simulink model "FS_FD1"  (R2021a)
settings: Solver=FixedStepAuto  StartTime=0.0  StopTime=inf  RelTol=1e-3
values from neighbouring files (symbols this model uses):
  waypoints = [0 0 0.089 0.468 1.137 1.887 2.636 3.385 4.128 4.865 5.608 6.345 ... (52 elements, 26x2)]    [waypoints_straight_corridor.mat]
undefined symbols (not defined in the file or in its folder): Angular, Linear
libraries: robotlib x5, robotalgslib x1, robotcorelib x1
settings Model: Creator=ACER  LastModifiedBy=tarun
settings OptimizationCC: EnhancedBackFolding=on  PassReuseOutputArgsAs=Individual arguments  ZeroExternalMemoryAtStartup=off  ZeroInternalMemoryAtStartup=off  MaxStackSize=64  OptimizeBlockOrder=speed  DifferentSizesBufferReuse=on  OptimizationCustomize=off  EfficientTunableParamExpr=on
settings DebuggingCC: ParameterTunabilityLossMsg=error
settings HardwareCC: ProdBitPerPointer=32  ProdBitPerSizeT=32  ProdBitPerPtrDiffT=32  ProdLargestAtomicFloat=None  ProdIntDivRoundTo=Undefined  ProdEndianess=Unspecified  ProdWordSize=32  ProdHWDeviceType=Generic->Unspecified (assume 32-bit Generic)
settings SFSimCC: MATLABDynamicMemAlloc=off
settings RTWCC: SystemTargetFile=ert.tlc  HardwareBoard=Robot Operating System (ROS)  TLCOptions="-aInlineSetEventsForThisBaseRateFcn=TLC_FALSE -aSuppressMultiTaskScheduler=TLC_FALSE  -aRateBasedStepFcn=0"  TemplateMakefile=ert_default_tmf  Toolchain=Catkin  TargetLang=C++
settings CodeAppCC: ForceParamTrailComments=on  IgnoreCustomStorageClasses=off  OperatorAnnotations=on  SimulinkDataObjDesc=on  SFDataObjDesc=on  InsertBlockDesc=on

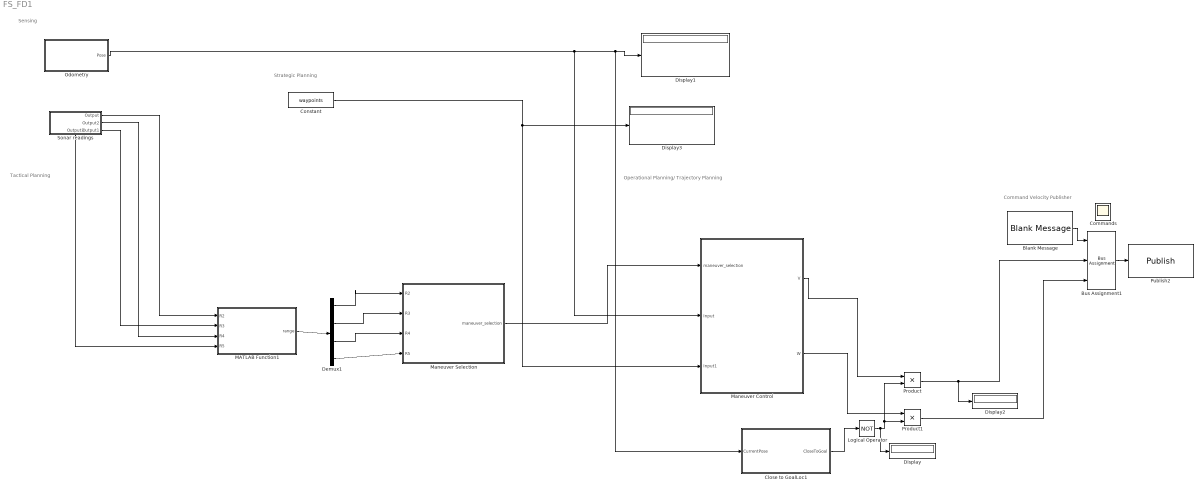
== system FS_FD1 ==
  note: Operational Planning/ Trajectory Planning
  note: Sensing
  note: Command Velocity Publisher
  note: Tactical Planning
  note: Strategic Planning
  Blank Message : robotlib/Blank Message  messageClass=Message  entityType=geometry_msgs/Twist  messageType=geometry_msgs/Twist  SampleTime=inf  legacyBusStruct=off
  Bus Assignment1 : BusAssignment  DialogController=Simulink.DDGSource_BusAssignment  AssignedSignals=Linear.X,Angular.Z
  Close to GoalLoc1 : Subsystem
  Commands : Scope  NumInputPorts=2
  Constant : Constant  Value=waypoints
  Demux1 : Demux
  Display{,1..3} (4 alike) : Display
  Logical Operator : Logic  Operator=NOT  AllPortsSameDT=off  OutDataTypeStr=boolean
  MATLAB Function1 : MATLAB Function  TreatAsAtomicUnit=on
  Maneuver Control : Subsystem
  Maneuver Selection : MATLAB Function  TreatAsAtomicUnit=on
  Odometry : Subsystem
  Product : Product
  Product1 : Product
  Publish2 : robotlib/Publish  topicSource=Select from ROS network  topic=/RosAria/cmd_vel  messageType=geometry_msgs/Twist  legacyBusStruct=off  messageQueueLength=105
  Sonar readings : Subsystem
      settings: PortSchema="{\"entries\":[{\"content\":{\"sides\":[{\"content\":{\"connectorIds\":[]},\"type\":\"ConnectorPlacement.EquallySpacedRectSide\",\"uuid\":\"cc9797a8-6551-4cc5-a464-2dfca9ae896a\"},{\"content\":{\"connectorIds\":[\"Out1\",\"Out2\",\"Out3\"],\"side\":\"RIGHT\"},\"type\":\"ConnectorPlacement.EquallySpacedRectSide\",\"uuid\":\"b2fd65e6-17ea-4988-b701-3713dcbefee6\"},{\"content\":{\"connectorIds\":[],\"side\":\"TOP\"},\"type\":\"ConnectorPlacement.EquallySpacedRectSide\",\"uuid\":\"23b966e9-18b1-4c56-9e9a-dc80dff313c9\"},{\"content\":{\"connectorIds\":[\"Out4\"],\"side\":\"BOTTOM\"},\"type\":\"ConnectorPlacement.EquallySpacedRectSide\",\"uuid\":\"b956123c-e71d-4c0e-8fc7-9c19c9412571\"}]},\"type\":\"ConnectorPlacement.EquallySpacedConnector\",\"uuid\":\"775a63bd-a867-418c-8661-cbcc6b0161f7\"}],\"packageUris\":[\"http://schema.mathworks.com/mf0/Connector/R2020b\"],\"version\":\"1.0\"}"
  wires:
  Constant/1 -> Maneuver Control/3(Input1), Display3/1
  Maneuver Control/1(V) -> Product/1
  Blank Message/1 -> Bus Assignment1/1
  Maneuver Selection/1(maneuver_selection) -> Maneuver Control/1(maneuver_selection)
  Bus Assignment1/1 -> Publish2/1
  Maneuver Control/2(W) -> Product1/1
  MATLAB Function1/1(range) -> Demux1/1
  Demux1/1 -> Maneuver Selection/1(R2)
  Demux1/2 -> Maneuver Selection/2(R3)
  Demux1/3 -> Maneuver Selection/3(R4)
  Demux1/4 -> Maneuver Selection/4(R5)
  Sonar readings/1(Output) -> MATLAB Function1/1(R2)
  Sonar readings/3(Output1) -> MATLAB Function1/2(R3)
  Sonar readings/2(Output2) -> MATLAB Function1/3(R4)
  Sonar readings/4(Output3) -> MATLAB Function1/4(R5)
  Odometry/1(Pose) -> Display1/1, Close to GoalLoc1/1(CurrentPose), Maneuver Control/2(Input)
  Close to GoalLoc1/1(CloseToGoal) -> Logical Operator/1
  Logical Operator/1 -> Display/1, Product1/2, Product/2
  Product/1 -> Display2/1, Bus Assignment1/2
  Product1/1 -> Bus Assignment1/3

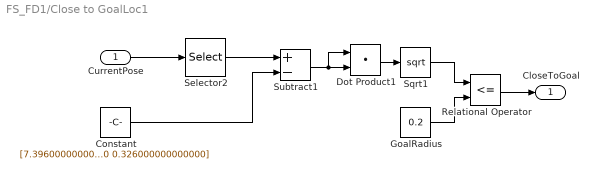
== system FS_FD1/Close to GoalLoc1 ==
  CurrentPose : Inport
  Constant : Constant  Value="[7.39600000000000\t0.326000000000000]"
  Dot Product1 : DotProduct  InputSameDT=on  OutDataTypeStr=Inherit: Inherit via internal rule
  GoalRadius : Constant  Value=0.2
  Relational Operator : RelationalOperator  Operator=<=  OutDataTypeStr=boolean  RndMeth=Simplest
  Selector2 : Selector  InputPortWidth=3  IndexOptions=Index vector (dialog)  Indices=[1 2]  OutputSizes=1
  Sqrt1 : Sqrt  SaturateOnIntegerOverflow=on
  Subtract1 : Sum  Inputs=+-
  CloseToGoal : Outport  VectorParamsAs1DForOutWhenUnconnected=off
  wires:
  Dot Product1/1 -> Sqrt1/1
  Subtract1/1 -> Dot Product1/1, Dot Product1/2
  Selector2/1 -> Subtract1/1
  Constant/1 -> Subtract1/2
  Sqrt1/1 -> Relational Operator/1
  GoalRadius/1 -> Relational Operator/2
  CurrentPose/1 -> Selector2/1
  Relational Operator/1 -> CloseToGoal/1

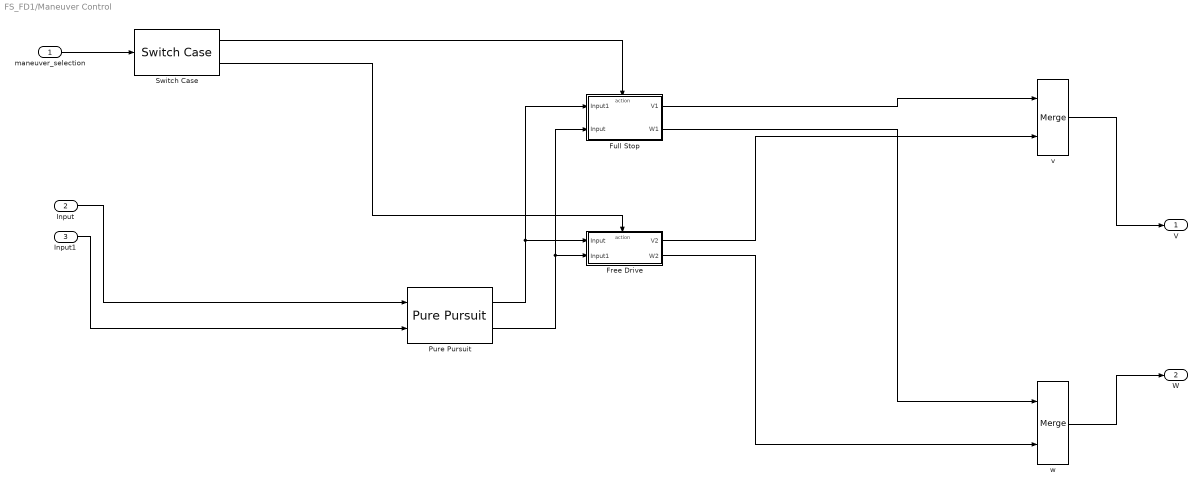
== system FS_FD1/Maneuver Control ==
  maneuver_selection : Inport
  Input : Inport  Port=2
  Input1 : Inport  Port=3
  Free Drive : Subsystem  TreatAsAtomicUnit=on
  Full Stop : Subsystem  TreatAsAtomicUnit=on
  Pure Pursuit : robotalgslib/Pure Pursuit  DesiredLinearVelocity=0.5  MaxAngularVelocity=0.8  LookaheadDistance=0.6  TargetDirPort=off  SimulateUsing=Code generation
  Switch Case : SwitchCase  CaseConditions={1,2}  ShowDefaultCase=off
  v : Merge
  w : Merge
  V : Outport
  W : Outport  Port=2
  wires:
  maneuver_selection/1 -> Switch Case/1
  Switch Case/1 -> Full Stop/Action
  Pure Pursuit/2 -> Full Stop/2(Input), Free Drive/2(Input1)
  Pure Pursuit/1 -> Full Stop/1(Input1), Free Drive/1(Input)
  Input1/1 -> Pure Pursuit/2
  Input/1 -> Pure Pursuit/1
  Free Drive/1(V2) -> v/2
  w/1 -> W/1
  v/1 -> V/1
  Switch Case/2 -> Free Drive/Action
  Full Stop/1(V1) -> v/1
  Full Stop/2(W1) -> w/1
  Free Drive/2(W2) -> w/2

== system FS_FD1/Odometry ==
  note: Generate a pose vector (x, y, theta) from X, Y, and quaternion data
  Bus Selector1 : BusSelector  OutputSignals=Pose.Pose.Position.X,Pose.Pose.Position.Y,Pose.Pose.Orientation.W,Pose.Pose.Orientation.X,Pose.Pose.Orientation.Y,Pose.Pose.Orientation.Z
  Coordinate Transformation Conversion : robotcorelib/Coordinate Transformation Conversion  InputRepresentation=Quaternion  InputEulerSequence=ZYX  ShowTrVecInputPort=on  OutputRepresentation=Euler Angles  OutputEulerSequence=ZYX  ShowTrVecOutputPort=on  SimulateUsing=Interpreted execution
      settings: SourceProductBaseCode=NV,RO,RR,UV
  Mux1 : Mux  Inputs=2
  Mux2 : Mux  Inputs=2
  Selector2 : Selector  InputPortWidth=3  IndexOptions=Index vector (dialog)  Indices=1  OutputSizes=1
  Subscribe1 : robotlib/Subscribe  topicSource=Select from ROS network  topic=/RosAria/pose  messageType=nav_msgs/Odometry  SampleTime=0.05  legacyBusStruct=off  messageQueueLength=51
  Terminator : Terminator
  Vector Concatenate : Concatenate  NumInputs=4
  Pose : Outport  VectorParamsAs1DForOutWhenUnconnected=off
  wires:
  Vector Concatenate/1 -> Coordinate Transformation Conversion/1
  Coordinate Transformation Conversion/1 -> Selector2/1
  Mux1/1 -> Mux2/1
  Selector2/1 -> Mux2/2
  Mux2/1 -> Pose/1
  Bus Selector1/6 -> Vector Concatenate/4  "<Z>"
  Bus Selector1/1 -> Mux1/1  "<X>"
  Bus Selector1/4 -> Vector Concatenate/2  "<X>"
  Bus Selector1/2 -> Mux1/2  "<Y>"
  Bus Selector1/5 -> Vector Concatenate/3  "<Y>"
  Subscribe1/2 -> Bus Selector1/1
  Bus Selector1/3 -> Vector Concatenate/1  "<W>"
  Subscribe1/1 -> Terminator/1

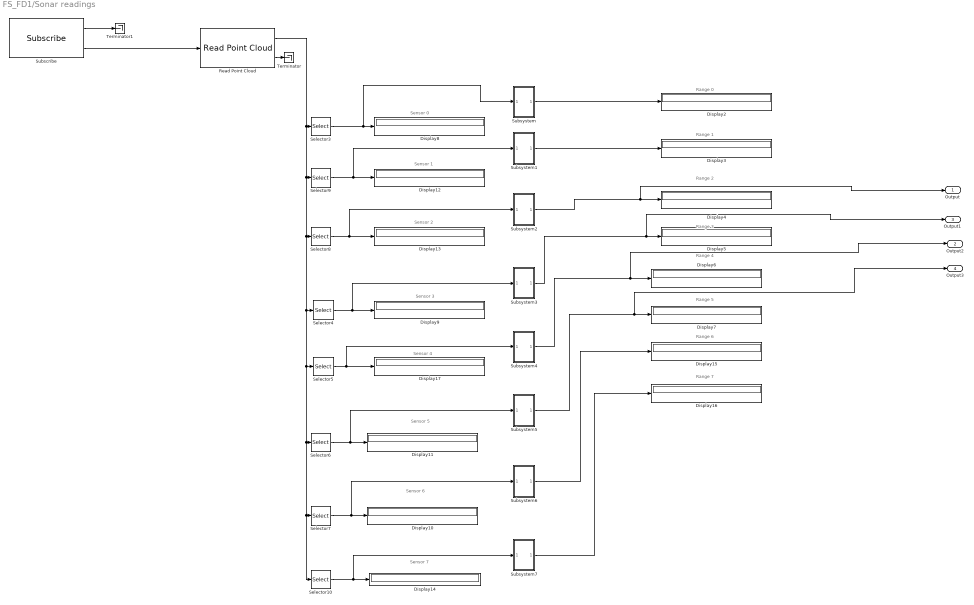
== system FS_FD1/Sonar readings ==
  note: Range 3
  note: Range 5
  note: Sensor 7
  note: Sensor 6
  note: Range 0
  note: Sensor 0
  note: Range 2
  note: Range 4
  note: Range 6
  note: Range 7
  note: Sensor 2
  note: Sensor 3
  note: Sensor 5
  note: Range 1
  note: Sensor 4
  note: Sensor 1
  Display{2..17} (16 alike) : Display
  Read Point Cloud : robotlib/Read Point Cloud  MaximumPointCloudSize=[8, 1]  PreserveStructure=off  ShowRGBOutput=off  ShowIntensityOutput=off  ShowErrorCodeOutput=on  VariableSizeOutputs=off
      settings: SourceProductBaseCode=RR
  Selector10 : Selector  NumberOfDimensions=2  InputPortWidth=6  IndexOptions=Starting index (dialog),Starting index (dialog)  Indices=8,1  OutputSizes=1,3
  Selector3 : Selector  NumberOfDimensions=2  InputPortWidth=6  IndexOptions=Starting index (dialog),Starting index (dialog)  Indices=1,1  OutputSizes=1,3
  Selector4 : Selector  NumberOfDimensions=2  InputPortWidth=6  IndexOptions=Starting index (dialog),Starting index (dialog)  Indices=4,1  OutputSizes=1,3
  Selector5 : Selector  NumberOfDimensions=2  InputPortWidth=6  IndexOptions=Starting index (dialog),Starting index (dialog)  Indices=5,1  OutputSizes=1,3
  Selector6 : Selector  NumberOfDimensions=2  InputPortWidth=6  IndexOptions=Starting index (dialog),Starting index (dialog)  Indices=6,1  OutputSizes=1,3
  Selector7 : Selector  NumberOfDimensions=2  InputPortWidth=6  IndexOptions=Starting index (dialog),Starting index (dialog)  Indices=7,1  OutputSizes=1,3
  Selector8 : Selector  NumberOfDimensions=2  InputPortWidth=6  IndexOptions=Starting index (dialog),Starting index (dialog)  Indices=3,1  OutputSizes=1,3
  Selector9 : Selector  NumberOfDimensions=2  InputPortWidth=6  IndexOptions=Starting index (dialog),Starting index (dialog)  Indices=2,1  OutputSizes=1,3
  Subscribe : robotlib/Subscribe  topicSource=Select from ROS network  topic=/RosAria/sonar_pointcloud2  messageType=sensor_msgs/PointCloud2  SampleTime=0.05  legacyBusStruct=off  messageQueueLength=1
  Subsystem : Subsystem
  Subsystem1 : Subsystem
  Subsystem2 : Subsystem
  Subsystem3 : Subsystem
  Subsystem4 : Subsystem
  Subsystem5 : Subsystem
  Subsystem6 : Subsystem
  Subsystem7 : Subsystem
  Terminator : Terminator
  Terminator1 : Terminator
  Output : Outport
  Output2 : Outport  Port=2
  Output1 : Outport  Port=3
  Output3 : Outport  Port=4
  wires:
  Subscribe/2 -> Read Point Cloud/1
  Subscribe/1 -> Terminator1/1
  Selector7/1 -> Subsystem6/1(In1), Display10/1
  Read Point Cloud/1 -> Selector3/1, Selector9/1, Selector8/1, Selector4/1, Selector5/1, Selector6/1, Selector10/1, Selector7/1
  Subsystem5/1(Output3) -> Output3/1, Display7/1
  Subsystem4/1(Output2) -> Output2/1, Display6/1
  Subsystem3/1(Output1) -> Output1/1, Display5/1
  Selector8/1 -> Subsystem2/1(In1), Display13/1
  Selector4/1 -> Subsystem3/1(In1), Display9/1
  Subsystem/1(Out1) -> Display2/1
  Selector9/1 -> Subsystem1/1(In1), Display12/1
  Selector5/1 -> Subsystem4/1(In1), Display17/1
  Read Point Cloud/2 -> Terminator/1
  Selector10/1 -> Subsystem7/1(In1), Display14/1
  Selector6/1 -> Subsystem5/1(In1), Display11/1
  Subsystem1/1(Out1) -> Display3/1
  Subsystem7/1(Out1) -> Display16/1
  Subsystem6/1(Out1) -> Display15/1
  Subsystem2/1(Output) -> Output/1, Display4/1
  Selector3/1 -> Display8/1, Subsystem/1(In1)

== system FS_FD1/Maneuver Control/Free Drive ==
  Input : Inport
  Input1 : Inport  Port=2
  Action Port : ActionPort  ActionPortLabel=case [ 2 ]:
  Gain : Gain
  Gain1 : Gain
  V2 : Outport
  W2 : Outport  Port=2
  wires:
  Input/1 -> Gain/1
  Gain/1 -> V2/1
  Input1/1 -> Gain1/1
  Gain1/1 -> W2/1

== system FS_FD1/Maneuver Control/Full Stop ==
  Input1 : Inport
  Input : Inport  Port=2
  Action Port : ActionPort  ActionPortLabel=case [ 1 ]:
  Gain : Gain  Gain=0
  Gain1 : Gain  Gain=0
  V1 : Outport
  W1 : Outport  Port=2
  wires:
  Gain/1 -> W1/1
  Input/1 -> Gain/1
  Input1/1 -> Gain1/1
  Gain1/1 -> V1/1

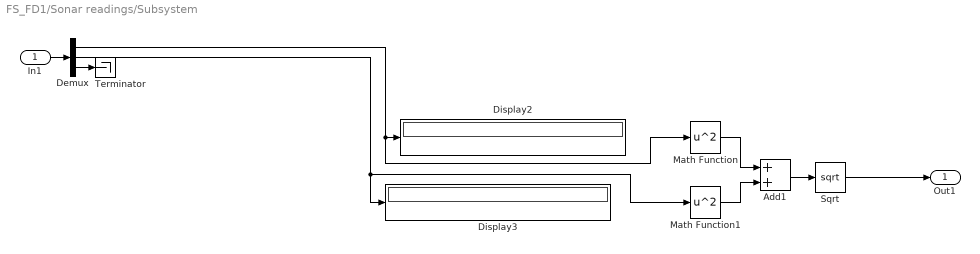
== system FS_FD1/Sonar readings/Subsystem ==
  In1 : Inport
  Add1 : Sum
  Demux : Demux  Outputs=3
  Display2 : Display
  Display3 : Display
  Math Function : Math  Operator=square  SaturateOnIntegerOverflow=on
  Math Function1 : Math  Operator=square  SaturateOnIntegerOverflow=on
  Sqrt : Sqrt  SaturateOnIntegerOverflow=on
  Terminator : Terminator
  Out1 : Outport
  wires:
  Math Function1/1 -> Add1/2
  Demux/1 -> Math Function/1, Display2/1
  In1/1 -> Demux/1
  Math Function/1 -> Add1/1
  Demux/2 -> Display3/1, Math Function1/1
  Sqrt/1 -> Out1/1
  Add1/1 -> Sqrt/1
  Demux/3 -> Terminator/1

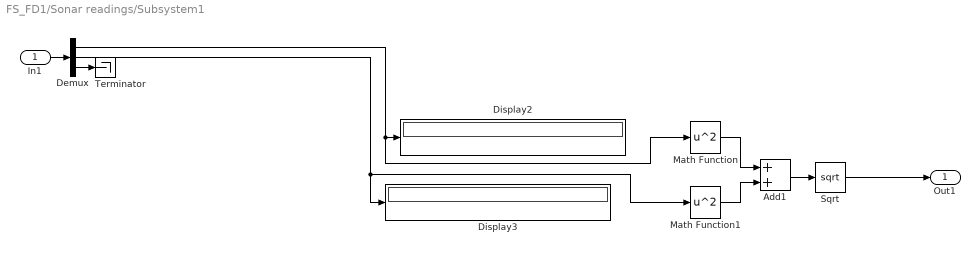
== system FS_FD1/Sonar readings/Subsystem1 ==
  In1 : Inport
  Add1 : Sum
  Demux : Demux  Outputs=3
  Display2 : Display
  Display3 : Display
  Math Function : Math  Operator=square  SaturateOnIntegerOverflow=on
  Math Function1 : Math  Operator=square  SaturateOnIntegerOverflow=on
  Sqrt : Sqrt  SaturateOnIntegerOverflow=on
  Terminator : Terminator
  Out1 : Outport
  wires:
  Math Function1/1 -> Add1/2
  Demux/1 -> Math Function/1, Display2/1
  In1/1 -> Demux/1
  Math Function/1 -> Add1/1
  Demux/2 -> Display3/1, Math Function1/1
  Sqrt/1 -> Out1/1
  Add1/1 -> Sqrt/1
  Demux/3 -> Terminator/1

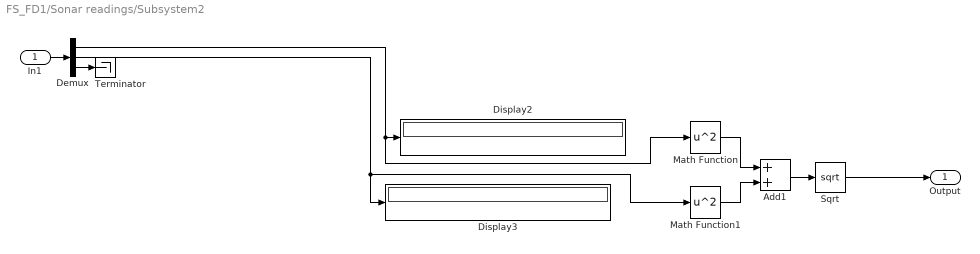
== system FS_FD1/Sonar readings/Subsystem2 ==
  In1 : Inport
  Add1 : Sum
  Demux : Demux  Outputs=3
  Display2 : Display
  Display3 : Display
  Math Function : Math  Operator=square  SaturateOnIntegerOverflow=on
  Math Function1 : Math  Operator=square  SaturateOnIntegerOverflow=on
  Sqrt : Sqrt  SaturateOnIntegerOverflow=on
  Terminator : Terminator
  Output : Outport
  wires:
  Math Function1/1 -> Add1/2
  Demux/1 -> Math Function/1, Display2/1
  In1/1 -> Demux/1
  Math Function/1 -> Add1/1
  Demux/2 -> Display3/1, Math Function1/1
  Sqrt/1 -> Output/1
  Add1/1 -> Sqrt/1
  Demux/3 -> Terminator/1

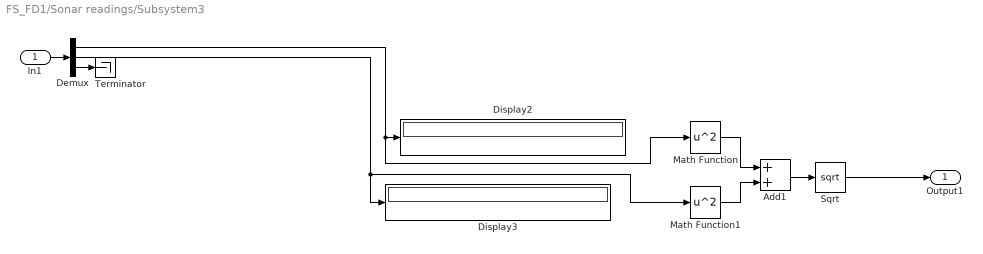
== system FS_FD1/Sonar readings/Subsystem3 ==
  In1 : Inport
  Add1 : Sum
  Demux : Demux  Outputs=3
  Display2 : Display
  Display3 : Display
  Math Function : Math  Operator=square  SaturateOnIntegerOverflow=on
  Math Function1 : Math  Operator=square  SaturateOnIntegerOverflow=on
  Sqrt : Sqrt  SaturateOnIntegerOverflow=on
  Terminator : Terminator
  Output1 : Outport
  wires:
  Math Function1/1 -> Add1/2
  Demux/1 -> Math Function/1, Display2/1
  In1/1 -> Demux/1
  Math Function/1 -> Add1/1
  Demux/2 -> Display3/1, Math Function1/1
  Sqrt/1 -> Output1/1
  Add1/1 -> Sqrt/1
  Demux/3 -> Terminator/1

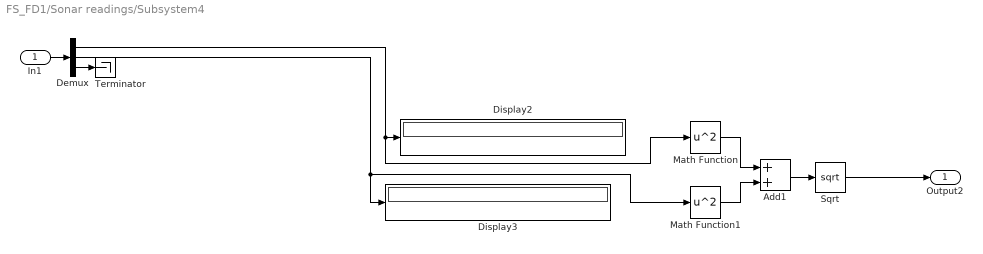
== system FS_FD1/Sonar readings/Subsystem4 ==
  In1 : Inport
  Add1 : Sum
  Demux : Demux  Outputs=3
  Display2 : Display
  Display3 : Display
  Math Function : Math  Operator=square  SaturateOnIntegerOverflow=on
  Math Function1 : Math  Operator=square  SaturateOnIntegerOverflow=on
  Sqrt : Sqrt  SaturateOnIntegerOverflow=on
  Terminator : Terminator
  Output2 : Outport
  wires:
  Math Function1/1 -> Add1/2
  Demux/1 -> Math Function/1, Display2/1
  In1/1 -> Demux/1
  Math Function/1 -> Add1/1
  Demux/2 -> Display3/1, Math Function1/1
  Sqrt/1 -> Output2/1
  Add1/1 -> Sqrt/1
  Demux/3 -> Terminator/1

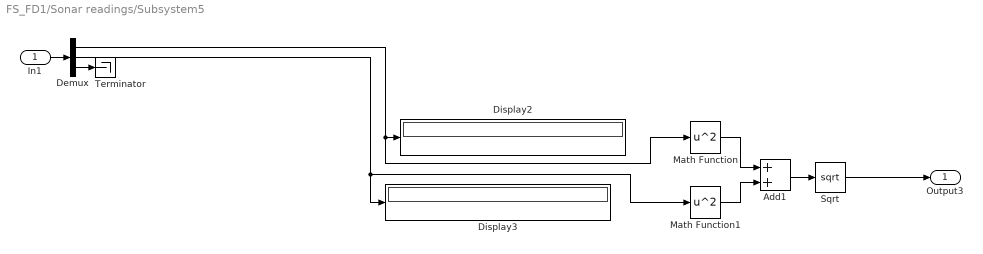
== system FS_FD1/Sonar readings/Subsystem5 ==
  In1 : Inport
  Add1 : Sum
  Demux : Demux  Outputs=3
  Display2 : Display
  Display3 : Display
  Math Function : Math  Operator=square  SaturateOnIntegerOverflow=on
  Math Function1 : Math  Operator=square  SaturateOnIntegerOverflow=on
  Sqrt : Sqrt  SaturateOnIntegerOverflow=on
  Terminator : Terminator
  Output3 : Outport
  wires:
  Math Function1/1 -> Add1/2
  Demux/1 -> Math Function/1, Display2/1
  In1/1 -> Demux/1
  Math Function/1 -> Add1/1
  Demux/2 -> Display3/1, Math Function1/1
  Sqrt/1 -> Output3/1
  Add1/1 -> Sqrt/1
  Demux/3 -> Terminator/1

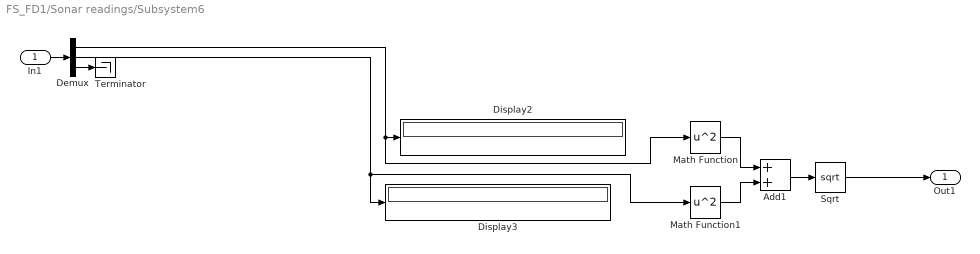
== system FS_FD1/Sonar readings/Subsystem6 ==
  In1 : Inport
  Add1 : Sum
  Demux : Demux  Outputs=3
  Display2 : Display
  Display3 : Display
  Math Function : Math  Operator=square  SaturateOnIntegerOverflow=on
  Math Function1 : Math  Operator=square  SaturateOnIntegerOverflow=on
  Sqrt : Sqrt  SaturateOnIntegerOverflow=on
  Terminator : Terminator
  Out1 : Outport
  wires:
  Math Function1/1 -> Add1/2
  Demux/1 -> Math Function/1, Display2/1
  In1/1 -> Demux/1
  Math Function/1 -> Add1/1
  Demux/2 -> Display3/1, Math Function1/1
  Sqrt/1 -> Out1/1
  Add1/1 -> Sqrt/1
  Demux/3 -> Terminator/1

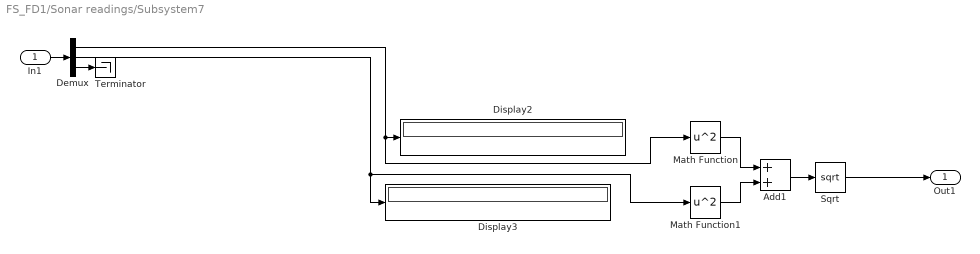
== system FS_FD1/Sonar readings/Subsystem7 ==
  In1 : Inport
  Add1 : Sum
  Demux : Demux  Outputs=3
  Display2 : Display
  Display3 : Display
  Math Function : Math  Operator=square  SaturateOnIntegerOverflow=on
  Math Function1 : Math  Operator=square  SaturateOnIntegerOverflow=on
  Sqrt : Sqrt  SaturateOnIntegerOverflow=on
  Terminator : Terminator
  Out1 : Outport
  wires:
  Math Function1/1 -> Add1/2
  Demux/1 -> Math Function/1, Display2/1
  In1/1 -> Demux/1
  Math Function/1 -> Add1/1
  Demux/2 -> Display3/1, Math Function1/1
  Sqrt/1 -> Out1/1
  Add1/1 -> Sqrt/1
  Demux/3 -> Terminator/1

== matlab function FS_FD1/Maneuver Selection ==
  data: R2 input; maneuver_selection output; R3 input; R4 input; R5 input
function maneuver_selection = fcn(R2,R3,R4,R5)
 if R2 < 1.5 || R3 < 1.5 || R4 < 1.5 || R5 < 1.5
    maneuver_selection = 1;
else 
     maneuver_selection = 2;
end

== matlab function FS_FD1/MATLAB Function1 ==
  data: range output; R2 input; R3 input; R4 input; R5 input
function range = sonarRanges(R2,R3,R4,R5)
range = [R2 R3 R4 R5];
end
